simulink model "MOBATSim"  (R2020b)
settings: Solver=FixedStepAuto  StartTime=0.0  StopTime=Sim_t  FixedStep=0.005  MinStep=0.01  RelTol=1e-2
undefined symbols (not defined in the file): FIBlock, FIBlockLib, meters, Sim_Ts, Vehicle_id, Vehicles
libraries: simulink x31, robotalgslib x11, drivingvehiclecontroller x11, mpcadaslib x1, pid_lib x1
(part 2 of 6)

== system MOBATSim/Vehicle Model 3 ==
  note: Perception
  note: Decision-Making
  note: Control
  Behavioural Planner : MATLABSystem  System=VehicleDrivingMode  Vehicle_id=Vehicle_id  SimulateUsing=Interpreted execution
      mask Type: VehicleDrivingMode
      mask Display:
      | image('MOBATSIM-Icon-Set_7- Behavioural Planner.png');
      | port_label('input',1,'vehicleDetected');
      | port_label('output',1,'SpeedReference');
      | port_label('output',2,'DistanceReference');
      | port_label('output',3,'LeadSpeed');
      | port_label('output',4,'DrivingMode');
      | port_label('output',5,'Dist2Stop');
      | port_label('output',6,'laneChange');
  Longitudinal and Lateral Controllers : Subsystem
  Safety Filter : Subsystem
  Transform to MOBATSim Coordinates : Subsystem
  Vehicle Model - Kinematic 3DOF Single Track : Subsystem  mask{Vehicle_id=Vehicle_id}
      mask prompts: Vehicle_id "Vehicle ID"
      mask Display: image('MOBATSIM-Icon-Set_13- VehicleModel.png'); % Use "Edit Image" on toolstrip to change.
  Vehicle Path Planner : MATLABSystem  System=VehiclePathPlanner_Astar  Vehicle_id=Vehicle_id  SimulateUsing=Interpreted execution
      mask Type: VehiclePathPlanner_Astar
      mask Display:
      | image('MOBATSIM-Icon-Set_8- Navigation.png');
      | port_label('input',1,'CommunicationIDs');
      | port_label('output',1,'waypointReached');
  Vehicle Sensors : MATLABSystem  System=VehicleSensors  Vehicle_id=Vehicle_id  Tsample=Sim_Ts  OffsetTime=0  SimulateUsing=Interpreted execution
      mask Type: VehicleSensors
      mask Display:
      | image('MOBATSIM-Icon-Set_4- Sensor.png');
      | port_label('output',1,'V2VcommIDs');
      | port_label('output',2,'vehicleDetected');
  Vehicle V2I Output : MATLABSystem  System=VehicleV2I_Out  Vehicle_id=Vehicle_id  SimulateUsing=Interpreted execution
      mask Type: VehicleV2I_Out
      mask Display:
      | image('MOBATSIM-Icon-Set_6- V2l.png');
      | port_label('input',1,'waypointReached');
      | port_label('output',1,'V2Idata');
  Position : Outport  VectorParamsAs1DForOutWhenUnconnected=off
  Orientation : Outport  Port=2  VectorParamsAs1DForOutWhenUnconnected=off
  Speed : Outport  Port=3  VectorParamsAs1DForOutWhenUnconnected=off
  V_Network_Out : Outport  Port=4  VectorParamsAs1DForOutWhenUnconnected=off
  wires:
  Vehicle Path Planner/1 -> Vehicle V2I Output/1
  Vehicle Sensors/1 -> Vehicle Path Planner/1
  Vehicle V2I Output/1 -> V_Network_Out/1
  Vehicle Sensors/2 -> Behavioural Planner/1
  Behavioural Planner/1 -> Longitudinal and Lateral Controllers/1(Speed Reference)
  Behavioural Planner/2 -> Longitudinal and Lateral Controllers/2(Inter Vehicular Distance)
  Behavioural Planner/3 -> Longitudinal and Lateral Controllers/3(Lead Speed)
  Behavioural Planner/4 -> Longitudinal and Lateral Controllers/4(drivingMode)
  Behavioural Planner/5 -> Longitudinal and Lateral Controllers/5(Dist2Stop)
  Transform to MOBATSim Coordinates/1(Position) -> Position/1
  Transform to MOBATSim Coordinates/2(Orientation) -> Orientation/1
  Vehicle Model - Kinematic 3DOF Single Track/2(xdot) -> Longitudinal and Lateral Controllers/7(Actual Speed), Speed/1
  Vehicle Model - Kinematic 3DOF Single Track/1(Pose) -> Longitudinal and Lateral Controllers/8(Actual Pose), Transform to MOBATSim Coordinates/1(Pose)
  Longitudinal and Lateral Controllers/1(ref Acc) -> Safety Filter/1(Reference Acceleration)
  Longitudinal and Lateral Controllers/2(ref Steering) -> Safety Filter/2(Reference Steering Angle)
  Safety Filter/1(Steering Angle Cmd) -> Vehicle Model - Kinematic 3DOF Single Track/1(WhlAngF)
  Safety Filter/2(Speed_input) -> Vehicle Model - Kinematic 3DOF Single Track/2(xdotin)
  Behavioural Planner/6 -> Longitudinal and Lateral Controllers/6(laneChange)

== system MOBATSim/Vehicle Model 4 ==
  note: Perception
  note: Decision-Making
  note: Control
  Behavioural Planner : MATLABSystem  System=VehicleDrivingMode  Vehicle_id=Vehicle_id  SimulateUsing=Interpreted execution
      mask Type: VehicleDrivingMode
      mask Display:
      | image('MOBATSIM-Icon-Set_7- Behavioural Planner.png');
      | port_label('input',1,'vehicleDetected');
      | port_label('output',1,'SpeedReference');
      | port_label('output',2,'DistanceReference');
      | port_label('output',3,'LeadSpeed');
      | port_label('output',4,'DrivingMode');
      | port_label('output',5,'Dist2Stop');
      | port_label('output',6,'laneChange');
  Longitudinal and Lateral Controllers : Subsystem
  Safety Filter : Subsystem
  Transform to MOBATSim Coordinates : Subsystem
  Vehicle Model - Kinematic 3DOF Single Track : Subsystem  mask{Vehicle_id=Vehicle_id}
      mask prompts: Vehicle_id "Vehicle ID"
      mask Display: image('MOBATSIM-Icon-Set_13- VehicleModel.png'); % Use "Edit Image" on toolstrip to change.
  Vehicle Path Planner : MATLABSystem  System=VehiclePathPlanner_Astar  Vehicle_id=Vehicle_id  SimulateUsing=Interpreted execution
      mask Type: VehiclePathPlanner_Astar
      mask Display:
      | image('MOBATSIM-Icon-Set_8- Navigation.png');
      | port_label('input',1,'CommunicationIDs');
      | port_label('output',1,'waypointReached');
  Vehicle Sensors : MATLABSystem  System=VehicleSensors  Vehicle_id=Vehicle_id  Tsample=Sim_Ts  OffsetTime=0  SimulateUsing=Interpreted execution
      mask Type: VehicleSensors
      mask Display:
      | image('MOBATSIM-Icon-Set_4- Sensor.png');
      | port_label('output',1,'V2VcommIDs');
      | port_label('output',2,'vehicleDetected');
  Vehicle V2I Output : MATLABSystem  System=VehicleV2I_Out  Vehicle_id=Vehicle_id  SimulateUsing=Interpreted execution
      mask Type: VehicleV2I_Out
      mask Display:
      | image('MOBATSIM-Icon-Set_6- V2l.png');
      | port_label('input',1,'waypointReached');
      | port_label('output',1,'V2Idata');
  Position : Outport  VectorParamsAs1DForOutWhenUnconnected=off
  Orientation : Outport  Port=2  VectorParamsAs1DForOutWhenUnconnected=off
  Speed : Outport  Port=3  VectorParamsAs1DForOutWhenUnconnected=off
  V_Network_Out : Outport  Port=4  VectorParamsAs1DForOutWhenUnconnected=off
  wires:
  Vehicle Path Planner/1 -> Vehicle V2I Output/1
  Vehicle Sensors/1 -> Vehicle Path Planner/1
  Vehicle V2I Output/1 -> V_Network_Out/1
  Vehicle Sensors/2 -> Behavioural Planner/1
  Behavioural Planner/1 -> Longitudinal and Lateral Controllers/1(Speed Reference)
  Behavioural Planner/2 -> Longitudinal and Lateral Controllers/2(Inter Vehicular Distance)
  Behavioural Planner/3 -> Longitudinal and Lateral Controllers/3(Lead Speed)
  Behavioural Planner/4 -> Longitudinal and Lateral Controllers/4(drivingMode)
  Behavioural Planner/5 -> Longitudinal and Lateral Controllers/5(Dist2Stop)
  Transform to MOBATSim Coordinates/1(Position) -> Position/1
  Transform to MOBATSim Coordinates/2(Orientation) -> Orientation/1
  Vehicle Model - Kinematic 3DOF Single Track/2(xdot) -> Longitudinal and Lateral Controllers/7(Actual Speed), Speed/1
  Vehicle Model - Kinematic 3DOF Single Track/1(Pose) -> Longitudinal and Lateral Controllers/8(Actual Pose), Transform to MOBATSim Coordinates/1(Pose)
  Longitudinal and Lateral Controllers/1(ref Acc) -> Safety Filter/1(Reference Acceleration)
  Longitudinal and Lateral Controllers/2(ref Steering) -> Safety Filter/2(Reference Steering Angle)
  Safety Filter/1(Steering Angle Cmd) -> Vehicle Model - Kinematic 3DOF Single Track/1(WhlAngF)
  Safety Filter/2(Speed_input) -> Vehicle Model - Kinematic 3DOF Single Track/2(xdotin)
  Behavioural Planner/6 -> Longitudinal and Lateral Controllers/6(laneChange)

== system MOBATSim/Vehicle Model 5 ==
  note: Perception
  note: Decision-Making
  note: Control
  Behavioural Planner : MATLABSystem  System=VehicleDrivingMode  Vehicle_id=Vehicle_id  SimulateUsing=Interpreted execution
      mask Type: VehicleDrivingMode
      mask Display:
      | image('MOBATSIM-Icon-Set_7- Behavioural Planner.png');
      | port_label('input',1,'vehicleDetected');
      | port_label('output',1,'SpeedReference');
      | port_label('output',2,'DistanceReference');
      | port_label('output',3,'LeadSpeed');
      | port_label('output',4,'DrivingMode');
      | port_label('output',5,'Dist2Stop');
      | port_label('output',6,'laneChange');
  Longitudinal and Lateral Controllers : Subsystem
  Safety Filter : Subsystem
  Transform to MOBATSim Coordinates : Subsystem
  Vehicle Model - Kinematic 3DOF Single Track : Subsystem  mask{Vehicle_id=Vehicle_id}
      mask prompts: Vehicle_id "Vehicle ID"
      mask Display: image('MOBATSIM-Icon-Set_13- VehicleModel.png'); % Use "Edit Image" on toolstrip to change.
  Vehicle Path Planner : MATLABSystem  System=VehiclePathPlanner_Astar  Vehicle_id=Vehicle_id  SimulateUsing=Interpreted execution
      mask Type: VehiclePathPlanner_Astar
      mask Display:
      | image('MOBATSIM-Icon-Set_8- Navigation.png');
      | port_label('input',1,'CommunicationIDs');
      | port_label('output',1,'waypointReached');
  Vehicle Sensors : MATLABSystem  System=VehicleSensors  Vehicle_id=Vehicle_id  Tsample=Sim_Ts  OffsetTime=0  SimulateUsing=Interpreted execution
      mask Type: VehicleSensors
      mask Display:
      | image('MOBATSIM-Icon-Set_4- Sensor.png');
      | port_label('output',1,'V2VcommIDs');
      | port_label('output',2,'vehicleDetected');
  Vehicle V2I Output : MATLABSystem  System=VehicleV2I_Out  Vehicle_id=Vehicle_id  SimulateUsing=Interpreted execution
      mask Type: VehicleV2I_Out
      mask Display:
      | image('MOBATSIM-Icon-Set_6- V2l.png');
      | port_label('input',1,'waypointReached');
      | port_label('output',1,'V2Idata');
  Position : Outport  VectorParamsAs1DForOutWhenUnconnected=off
  Orientation : Outport  Port=2  VectorParamsAs1DForOutWhenUnconnected=off
  Speed : Outport  Port=3  VectorParamsAs1DForOutWhenUnconnected=off
  V_Network_Out : Outport  Port=4  VectorParamsAs1DForOutWhenUnconnected=off
  wires:
  Vehicle Path Planner/1 -> Vehicle V2I Output/1
  Vehicle Sensors/1 -> Vehicle Path Planner/1
  Vehicle V2I Output/1 -> V_Network_Out/1
  Vehicle Sensors/2 -> Behavioural Planner/1
  Behavioural Planner/1 -> Longitudinal and Lateral Controllers/1(Speed Reference)
  Behavioural Planner/2 -> Longitudinal and Lateral Controllers/2(Inter Vehicular Distance)
  Behavioural Planner/3 -> Longitudinal and Lateral Controllers/3(Lead Speed)
  Behavioural Planner/4 -> Longitudinal and Lateral Controllers/4(drivingMode)
  Behavioural Planner/5 -> Longitudinal and Lateral Controllers/5(Dist2Stop)
  Transform to MOBATSim Coordinates/1(Position) -> Position/1
  Transform to MOBATSim Coordinates/2(Orientation) -> Orientation/1
  Vehicle Model - Kinematic 3DOF Single Track/2(xdot) -> Longitudinal and Lateral Controllers/7(Actual Speed), Speed/1
  Vehicle Model - Kinematic 3DOF Single Track/1(Pose) -> Longitudinal and Lateral Controllers/8(Actual Pose), Transform to MOBATSim Coordinates/1(Pose)
  Longitudinal and Lateral Controllers/1(ref Acc) -> Safety Filter/1(Reference Acceleration)
  Longitudinal and Lateral Controllers/2(ref Steering) -> Safety Filter/2(Reference Steering Angle)
  Safety Filter/1(Steering Angle Cmd) -> Vehicle Model - Kinematic 3DOF Single Track/1(WhlAngF)
  Safety Filter/2(Speed_input) -> Vehicle Model - Kinematic 3DOF Single Track/2(xdotin)
  Behavioural Planner/6 -> Longitudinal and Lateral Controllers/6(laneChange)

== system MOBATSim/Vehicle Model 6 ==
  note: Perception
  note: Decision-Making
  note: Control
  Behavioural Planner : MATLABSystem  System=VehicleDrivingMode  Vehicle_id=Vehicle_id  SimulateUsing=Interpreted execution
      mask Type: VehicleDrivingMode
      mask Display:
      | image('MOBATSIM-Icon-Set_7- Behavioural Planner.png');
      | port_label('input',1,'vehicleDetected');
      | port_label('output',1,'SpeedReference');
      | port_label('output',2,'DistanceReference');
      | port_label('output',3,'LeadSpeed');
      | port_label('output',4,'DrivingMode');
      | port_label('output',5,'Dist2Stop');
      | port_label('output',6,'laneChange');
  FIBlock : Subsystem  AncestorBlock=FIBlockLib/FIBlock  TreatAsAtomicUnit=on  mask(Fault Injector Block){FIBlockName=1, FInjEnable=on, FaultType=Noise, FaultValue=20, FaultEvent=Deterministic, EventValue=0, FaultEffect=Constant time, EffectValue=4.2}
      mask prompts: FIBlockName "Number of the FI block instance (e.i. 'name' of the fault injector)"; FInjEnable "Turn on the fault injection for this block"; FaultType "Fault type"; FaultValue "Fault value (boundaries, %)"; FaultEvent "Fault injection method"; EventValue "Event value (s)"; FaultEffect "Fault injection effect"; EffectValue "Effect value (s)"
      mask help:
      | This block allows to conduct a fault injection experiment (refer to help if needed).
      | Specify:
      | - name of the block instance.
      | - type of fault: Stuck-at, Package drop, Bias/Offset, Bit flips, Time delay, Noise.
      | - fault event: Failure probability, Mean Time to Failure, Failure Rate Distribution, Deterministic.
      | - fault effect: Once, Constant time, Infinite time, Mean Time to Repair.
      mask init: same as MOBATSim/Vehicle Model 2/FIBlock1
      mask Help:
      | Failure rate distribution is not supported yet!
      | Bit flips, Time delay, and Noise faults may have some bugs :D
      | In different FIBlock instances, the 'name' of the block in GUI must be different (must be an integer number).
      | 
      | Please refer to a comprehensive article regarding the FIBLock: https://flatag.tech/fiblock.html
      | Please cite as: "Fabarisov, T. et al. "Model-based Fault Injection Experiments for the Safety Analysis of Exoskeleton System." Proceedings of the 30th European Safety and Reliability Conference and the 15th Probabilistic Safety Assessment and Management Conference, 2020."
      | 
      | This block allows to conduct a fault injection experiment.
      | Specify:
      | 1) number of the block instance (e.i. 'name' of the fault injector, name shall be unique).
      | 
      | 2) type of fault:
      | - Stuck-at. The block output stays constant, preserving the latest correct value before the error occurrence.
      | - Package drop. The correct output is replaced by the specified Value, emulating a package drop.
      | - Bias/Offset . The defined positive or negative Bias value is added to the block output.
      | - Noise. A random noise value is added. The Boundaries are defined as the percentage of the correct value.
      | - Time delay. A delay is introduced into the signal. During the delay the value is zero.
      | - Bit flips. The defined Number of bits are inverted in the binary representation of the correct value.
      | 
      | 3) fault event:
      | - Failure probability. Errors are injected based on the constant Failure probability for each execution of the block function.
      | - Mean Time to Failure. Errors are injected according to the specified MTTF. Normal distribution.
      | - Deterministic. Уrrors are injected at specific time step.
      | 
      | 4) fault effect:
      | - Once. An error appears only one time during a simulation.
      | - Constant time. The block produces erroneous output during the specified Time period.
      | - Infinite time. The block produces erroneous output until the end of the simulation.
      | - Mean Time to Repair. Normally distributed MTTR regulates the time of the error effect.
      | 
      | FIBlock also provide, what we call, a chained fault injection.
      | Second output of the FIBlock emits a trigger flag.
      | This output signal could be connected to the second input of the FIBlock.
      | In case of the fault injection, this signal will force trigger fault injectionin second FIBlock.
      | 
      | FIBlock supports a base Workspace variables as input in the GUI parameters.
      | 
      | Made By Tagir Fabarisov, TU Dresden 2020
      mask TypeOptions FaultType: Stuck-at | Package drop | Bias/Offset | Bit flips | Time delay | Noise
      mask TypeOptions FaultEvent: Failure probability | Mean Time To Failure | Deterministic
      mask TypeOptions FaultEffect: Once | Constant time | Infinite time | Mean Time To Repair
      mask DialogControl FInjEnable Tooltip: If ticked, then this FIBlock will inject faults
      mask DialogControl Container8 Prompt: Fault type
      mask DialogControl FaultType Tooltip: Specify a type of fault that will be injected
      mask DialogControl FaultTypeDesc Prompt: A random noise value is added. The Boundaries are defined as the percentage of the correct value.
      mask DialogControl Container3 Prompt: Fault injection method
      mask DialogControl Container6 Prompt: Event
      mask DialogControl FaultEvent Tooltip: Specify when fault will be injected
      mask DialogControl FaultEventDesc Prompt: Errors are injected at the specified time
      mask DialogControl Container7 Prompt: Effect
      mask DialogControl FaultEffect Tooltip: Specify how long fault will be injected
      mask DialogControl FaultEffectDesc Prompt: The block produces erroneous output during the specified Time period.
      mask Display:
      | warning off;
      | color('red');
      | a = FaultType;
      | if a == "Sensor: Stuck-at fault"
      |     color('black');
      |     x = linspace(-pi,pi);
      |     y = sin(x);
      |     plot(x,y);
      |     color('red');
      |     disp('        ↯');
      |     x = [-0.7 2];
      |     y = [-0.7 -0.7];
      |     plot(x,y);
      | elseif a == "Network: Package drop"
      |     color('black');
      |     x = linspace(-pi,pi);
      |     y = sin(x);
      |     plot(x,y);
      |     color('red');
      |     disp('        ↯');
      |     x = [-0.7 -0.7];
      |     y = [-0.7 0];
      |     plot(x,y);
      |     x = [-0.7 1];
      |     y = [0 0];
      |     plot(x,y);
      | elseif a == "Sensor: Offset"
      |     color('black');
      |     x1 = linspace(-pi,pi);
      |     y1 = sin(x1)-0.5;
      |     plot(x1,y1);
      |     color('red');
      |     disp('        ↯');
      |     x2 = linspace(0,pi);
      |     y2 = sin(x2);
      |     plot(x2,y2);
      |     x = [0 0];
      |     y = [-0.5 0];
      |     plot(x,y);
      | elseif a == "Hardware: Bit flips"
      |     color('black');
      |     disp('10101010');
      |     color('red');
      |     disp('    0↯');
      | elseif a == "Network: Time delay"
      |     color('black');
      |     x1 = linspace(-pi,pi);
      |     y1 = sin(x1);
      |     plot(x1,y1);
      |     color('red');
      |     disp('        ↯');
      |     x2 = linspace(0,pi);
      |     y2 = sin(x2-0.5);
      |     plot(x2,y2);
      |     x = [0 -0.4];
      |     y = [-0.5 -0.5];
      |     plot(x,y);
      | elseif a == "Sensor: Noise"
      |     color('black');
      |     x1 = linspace(-pi,pi);
      |     y1 = sin(x1);
      |     plot(x1,y1);
      |     color('red');
      |     disp('        ↯');
      |     x = linspace(-pi/8,pi/8,10);
      |     y = sin(x);
      |     for yc = 1:length(y)
      |         d = randi([-2,2])/5;
      |         y(yc) = y(yc) + d;
      |     end
      |     plot(x,y);
      | else
      |     color('red');
      |     disp('Set up Fault Injector!');
      | %Bit flips
      | %Time delay
      | %Noise
      | end
      | warning on;
  FIBlock1 : Subsystem  AncestorBlock=FIBlockLib/FIBlock  TreatAsAtomicUnit=on  mask(Fault Injector Block){FIBlockName=2, FInjEnable=on, FaultType=Noise, FaultValue=20, FaultEvent=Deterministic, EventValue=0, FaultEffect=Constant time, EffectValue=4.2}
      mask prompts: FIBlockName "Number of the FI block instance (e.i. 'name' of the fault injector)"; FInjEnable "Turn on the fault injection for this block"; FaultType "Fault type"; FaultValue "Fault value (boundaries, %)"; FaultEvent "Fault injection method"; EventValue "Event value (s)"; FaultEffect "Fault injection effect"; EffectValue "Effect value (s)"
      mask help:
      | This block allows to conduct a fault injection experiment (refer to help if needed).
      | Specify:
      | - name of the block instance.
      | - type of fault: Stuck-at, Package drop, Bias/Offset, Bit flips, Time delay, Noise.
      | - fault event: Failure probability, Mean Time to Failure, Failure Rate Distribution, Deterministic.
      | - fault effect: Once, Constant time, Infinite time, Mean Time to Repair.
      mask init: same as MOBATSim/Vehicle Model 2/FIBlock1
      mask Help:
      | Failure rate distribution is not supported yet!
      | Bit flips, Time delay, and Noise faults may have some bugs :D
      | In different FIBlock instances, the 'name' of the block in GUI must be different (must be an integer number).
      | 
      | Please refer to a comprehensive article regarding the FIBLock: https://flatag.tech/fiblock.html
      | Please cite as: "Fabarisov, T. et al. "Model-based Fault Injection Experiments for the Safety Analysis of Exoskeleton System." Proceedings of the 30th European Safety and Reliability Conference and the 15th Probabilistic Safety Assessment and Management Conference, 2020."
      | 
      | This block allows to conduct a fault injection experiment.
      | Specify:
      | 1) number of the block instance (e.i. 'name' of the fault injector, name shall be unique).
      | 
      | 2) type of fault:
      | - Stuck-at. The block output stays constant, preserving the latest correct value before the error occurrence.
      | - Package drop. The correct output is replaced by the specified Value, emulating a package drop.
      | - Bias/Offset . The defined positive or negative Bias value is added to the block output.
      | - Noise. A random noise value is added. The Boundaries are defined as the percentage of the correct value.
      | - Time delay. A delay is introduced into the signal. During the delay the value is zero.
      | - Bit flips. The defined Number of bits are inverted in the binary representation of the correct value.
      | 
      | 3) fault event:
      | - Failure probability. Errors are injected based on the constant Failure probability for each execution of the block function.
      | - Mean Time to Failure. Errors are injected according to the specified MTTF. Normal distribution.
      | - Deterministic. Уrrors are injected at specific time step.
      | 
      | 4) fault effect:
      | - Once. An error appears only one time during a simulation.
      | - Constant time. The block produces erroneous output during the specified Time period.
      | - Infinite time. The block produces erroneous output until the end of the simulation.
      | - Mean Time to Repair. Normally distributed MTTR regulates the time of the error effect.
      | 
      | FIBlock also provide, what we call, a chained fault injection.
      | Second output of the FIBlock emits a trigger flag.
      | This output signal could be connected to the second input of the FIBlock.
      | In case of the fault injection, this signal will force trigger fault injectionin second FIBlock.
      | 
      | FIBlock supports a base Workspace variables as input in the GUI parameters.
      | 
      | Made By Tagir Fabarisov, TU Dresden 2020
      mask TypeOptions FaultType: Stuck-at | Package drop | Bias/Offset | Bit flips | Time delay | Noise
      mask TypeOptions FaultEvent: Failure probability | Mean Time To Failure | Deterministic
      mask TypeOptions FaultEffect: Once | Constant time | Infinite time | Mean Time To Repair
      mask DialogControl FInjEnable Tooltip: If ticked, then this FIBlock will inject faults
      mask DialogControl Container8 Prompt: Fault type
      mask DialogControl FaultType Tooltip: Specify a type of fault that will be injected
      mask DialogControl FaultTypeDesc Prompt: A random noise value is added. The Boundaries are defined as the percentage of the correct value.
      mask DialogControl Container3 Prompt: Fault injection method
      mask DialogControl Container6 Prompt: Event
      mask DialogControl FaultEvent Tooltip: Specify when fault will be injected
      mask DialogControl FaultEventDesc Prompt: Errors are injected at the specified time
      mask DialogControl Container7 Prompt: Effect
      mask DialogControl FaultEffect Tooltip: Specify how long fault will be injected
      mask DialogControl FaultEffectDesc Prompt: The block produces erroneous output during the specified Time period.
      mask Display:
      | warning off;
      | color('red');
      | a = FaultType;
      | if a == "Sensor: Stuck-at fault"
      |     color('black');
      |     x = linspace(-pi,pi);
      |     y = sin(x);
      |     plot(x,y);
      |     color('red');
      |     disp('        ↯');
      |     x = [-0.7 2];
      |     y = [-0.7 -0.7];
      |     plot(x,y);
      | elseif a == "Network: Package drop"
      |     color('black');
      |     x = linspace(-pi,pi);
      |     y = sin(x);
      |     plot(x,y);
      |     color('red');
      |     disp('        ↯');
      |     x = [-0.7 -0.7];
      |     y = [-0.7 0];
      |     plot(x,y);
      |     x = [-0.7 1];
      |     y = [0 0];
      |     plot(x,y);
      | elseif a == "Sensor: Offset"
      |     color('black');
      |     x1 = linspace(-pi,pi);
      |     y1 = sin(x1)-0.5;
      |     plot(x1,y1);
      |     color('red');
      |     disp('        ↯');
      |     x2 = linspace(0,pi);
      |     y2 = sin(x2);
      |     plot(x2,y2);
      |     x = [0 0];
      |     y = [-0.5 0];
      |     plot(x,y);
      | elseif a == "Hardware: Bit flips"
      |     color('black');
      |     disp('10101010');
      |     color('red');
      |     disp('    0↯');
      | elseif a == "Network: Time delay"
      |     color('black');
      |     x1 = linspace(-pi,pi);
      |     y1 = sin(x1);
      |     plot(x1,y1);
      |     color('red');
      |     disp('        ↯');
      |     x2 = linspace(0,pi);
      |     y2 = sin(x2-0.5);
      |     plot(x2,y2);
      |     x = [0 -0.4];
      |     y = [-0.5 -0.5];
      |     plot(x,y);
      | elseif a == "Sensor: Noise"
      |     color('black');
      |     x1 = linspace(-pi,pi);
      |     y1 = sin(x1);
      |     plot(x1,y1);
      |     color('red');
      |     disp('        ↯');
      |     x = linspace(-pi/8,pi/8,10);
      |     y = sin(x);
      |     for yc = 1:length(y)
      |         d = randi([-2,2])/5;
      |         y(yc) = y(yc) + d;
      |     end
      |     plot(x,y);
      | else
      |     color('red');
      |     disp('Set up Fault Injector!');
      | %Bit flips
      | %Time delay
      | %Noise
      | end
      | warning on;
  Longitudinal and Lateral Controllers : Subsystem
  Pulse Generator : DiscretePulseGenerator  PulseType=Time based  Period=10  PulseWidth=5
  Pulse Generator1 : DiscretePulseGenerator  PulseType=Time based  Period=10  PulseWidth=5
  Safety Filter : Subsystem
  Transform to MOBATSim Coordinates : Subsystem
  Vehicle Model - Kinematic 3DOF Single Track : Subsystem  mask{Vehicle_id=Vehicle_id}
      mask prompts: Vehicle_id "Vehicle ID"
      mask Display: image('MOBATSIM-Icon-Set_13- VehicleModel.png'); % Use "Edit Image" on toolstrip to change.
  Vehicle Path Planner : MATLABSystem  System=VehiclePathPlanner_Astar  Vehicle_id=Vehicle_id  SimulateUsing=Interpreted execution
      mask Type: VehiclePathPlanner_Astar
      mask Display:
      | image('MOBATSIM-Icon-Set_8- Navigation.png');
      | port_label('input',1,'CommunicationIDs');
      | port_label('output',1,'waypointReached');
  Vehicle Sensors : MATLABSystem  System=VehicleSensors  Vehicle_id=Vehicle_id  Tsample=Sim_Ts  OffsetTime=0  SimulateUsing=Interpreted execution
      mask Type: VehicleSensors
      mask Display:
      | image('MOBATSIM-Icon-Set_4- Sensor.png');
      | port_label('output',1,'V2VcommIDs');
      | port_label('output',2,'vehicleDetected');
  Vehicle V2I Output : MATLABSystem  System=VehicleV2I_Out  Vehicle_id=Vehicle_id  SimulateUsing=Interpreted execution
      mask Type: VehicleV2I_Out
      mask Display:
      | image('MOBATSIM-Icon-Set_6- V2l.png');
      | port_label('input',1,'waypointReached');
      | port_label('output',1,'V2Idata');
  Position : Outport  VectorParamsAs1DForOutWhenUnconnected=off
  Orientation : Outport  Port=2  VectorParamsAs1DForOutWhenUnconnected=off
  Speed : Outport  Port=3  VectorParamsAs1DForOutWhenUnconnected=off
  V_Network_Out : Outport  Port=4  VectorParamsAs1DForOutWhenUnconnected=off
  wires:
  Vehicle Path Planner/1 -> Vehicle V2I Output/1
  Vehicle Sensors/1 -> Vehicle Path Planner/1
  Vehicle V2I Output/1 -> V_Network_Out/1
  Vehicle Sensors/2 -> Behavioural Planner/1
  Behavioural Planner/3 -> Longitudinal and Lateral Controllers/3(Lead Speed)
  Behavioural Planner/4 -> Longitudinal and Lateral Controllers/4(drivingMode)
  Behavioural Planner/5 -> Longitudinal and Lateral Controllers/5(Dist2Stop)
  Transform to MOBATSim Coordinates/1(Position) -> Position/1
  Transform to MOBATSim Coordinates/2(Orientation) -> Orientation/1
  Vehicle Model - Kinematic 3DOF Single Track/2(xdot) -> Longitudinal and Lateral Controllers/7(Actual Speed), Speed/1
  Vehicle Model - Kinematic 3DOF Single Track/1(Pose) -> Longitudinal and Lateral Controllers/8(Actual Pose), Transform to MOBATSim Coordinates/1(Pose)
  Longitudinal and Lateral Controllers/1(ref Acc) -> Safety Filter/1(Reference Acceleration)
  Longitudinal and Lateral Controllers/2(ref Steering) -> Safety Filter/2(Reference Steering Angle)
  Safety Filter/1(Steering Angle Cmd) -> Vehicle Model - Kinematic 3DOF Single Track/1(WhlAngF)
  Safety Filter/2(Speed_input) -> Vehicle Model - Kinematic 3DOF Single Track/2(xdotin)
  Behavioural Planner/6 -> Longitudinal and Lateral Controllers/6(laneChange)
  Behavioural Planner/1 -> FIBlock/1(Idata)
  FIBlock/1(Fdata) -> Longitudinal and Lateral Controllers/1(Speed Reference)
  Behavioural Planner/2 -> FIBlock1/1(Idata)
  FIBlock1/1(Fdata) -> Longitudinal and Lateral Controllers/2(Inter Vehicular Distance)
  Pulse Generator1/1 -> FIBlock/2(Iflag)
  Pulse Generator/1 -> FIBlock1/2(Iflag)

== system MOBATSim/Vehicle Model 7 ==
  note: Perception
  note: Decision-Making
  note: Control
  Behavioural Planner : MATLABSystem  System=VehicleDrivingMode  Vehicle_id=Vehicle_id  SimulateUsing=Interpreted execution
      mask Type: VehicleDrivingMode
      mask Display:
      | image('MOBATSIM-Icon-Set_7- Behavioural Planner.png');
      | port_label('input',1,'vehicleDetected');
      | port_label('output',1,'SpeedReference');
      | port_label('output',2,'DistanceReference');
      | port_label('output',3,'LeadSpeed');
      | port_label('output',4,'DrivingMode');
      | port_label('output',5,'Dist2Stop');
      | port_label('output',6,'laneChange');
  Longitudinal and Lateral Controllers : Subsystem
  Safety Filter : Subsystem
  Transform to MOBATSim Coordinates : Subsystem
  Vehicle Model - Kinematic 3DOF Single Track : Subsystem  mask{Vehicle_id=Vehicle_id}
      mask prompts: Vehicle_id "Vehicle ID"
      mask Display: image('MOBATSIM-Icon-Set_13- VehicleModel.png'); % Use "Edit Image" on toolstrip to change.
  Vehicle Path Planner : MATLABSystem  System=VehiclePathPlanner_Astar  Vehicle_id=Vehicle_id  SimulateUsing=Interpreted execution
      mask Type: VehiclePathPlanner_Astar
      mask Display:
      | image('MOBATSIM-Icon-Set_8- Navigation.png');
      | port_label('input',1,'CommunicationIDs');
      | port_label('output',1,'waypointReached');
  Vehicle Sensors : MATLABSystem  System=VehicleSensors  Vehicle_id=Vehicle_id  Tsample=Sim_Ts  OffsetTime=0  SimulateUsing=Interpreted execution
      mask Type: VehicleSensors
      mask Display:
      | image('MOBATSIM-Icon-Set_4- Sensor.png');
      | port_label('output',1,'V2VcommIDs');
      | port_label('output',2,'vehicleDetected');
  Vehicle V2I Output : MATLABSystem  System=VehicleV2I_Out  Vehicle_id=Vehicle_id  SimulateUsing=Interpreted execution
      mask Type: VehicleV2I_Out
      mask Display:
      | image('MOBATSIM-Icon-Set_6- V2l.png');
      | port_label('input',1,'waypointReached');
      | port_label('output',1,'V2Idata');
  Position : Outport  VectorParamsAs1DForOutWhenUnconnected=off
  Orientation : Outport  Port=2  VectorParamsAs1DForOutWhenUnconnected=off
  Speed : Outport  Port=3  VectorParamsAs1DForOutWhenUnconnected=off
  V_Network_Out : Outport  Port=4  VectorParamsAs1DForOutWhenUnconnected=off
  wires:
  Vehicle Path Planner/1 -> Vehicle V2I Output/1
  Vehicle Sensors/1 -> Vehicle Path Planner/1
  Vehicle V2I Output/1 -> V_Network_Out/1
  Vehicle Sensors/2 -> Behavioural Planner/1
  Behavioural Planner/1 -> Longitudinal and Lateral Controllers/1(Speed Reference)
  Behavioural Planner/2 -> Longitudinal and Lateral Controllers/2(Inter Vehicular Distance)
  Behavioural Planner/3 -> Longitudinal and Lateral Controllers/3(Lead Speed)
  Behavioural Planner/4 -> Longitudinal and Lateral Controllers/4(drivingMode)
  Behavioural Planner/5 -> Longitudinal and Lateral Controllers/5(Dist2Stop)
  Transform to MOBATSim Coordinates/1(Position) -> Position/1
  Transform to MOBATSim Coordinates/2(Orientation) -> Orientation/1
  Vehicle Model - Kinematic 3DOF Single Track/2(xdot) -> Longitudinal and Lateral Controllers/7(Actual Speed), Speed/1
  Vehicle Model - Kinematic 3DOF Single Track/1(Pose) -> Longitudinal and Lateral Controllers/8(Actual Pose), Transform to MOBATSim Coordinates/1(Pose)
  Longitudinal and Lateral Controllers/1(ref Acc) -> Safety Filter/1(Reference Acceleration)
  Longitudinal and Lateral Controllers/2(ref Steering) -> Safety Filter/2(Reference Steering Angle)
  Safety Filter/1(Steering Angle Cmd) -> Vehicle Model - Kinematic 3DOF Single Track/1(WhlAngF)
  Safety Filter/2(Speed_input) -> Vehicle Model - Kinematic 3DOF Single Track/2(xdotin)
  Behavioural Planner/6 -> Longitudinal and Lateral Controllers/6(laneChange)

== system MOBATSim/Vehicle Model 8 ==
  note: Perception
  note: Decision-Making
  note: Control
  Behavioural Planner : MATLABSystem  System=VehicleDrivingMode  Vehicle_id=Vehicle_id  SimulateUsing=Interpreted execution
      mask Type: VehicleDrivingMode
      mask Display:
      | image('MOBATSIM-Icon-Set_7- Behavioural Planner.png');
      | port_label('input',1,'vehicleDetected');
      | port_label('output',1,'SpeedReference');
      | port_label('output',2,'DistanceReference');
      | port_label('output',3,'LeadSpeed');
      | port_label('output',4,'DrivingMode');
      | port_label('output',5,'Dist2Stop');
      | port_label('output',6,'laneChange');
  Longitudinal and Lateral Controllers : Subsystem
  Safety Filter : Subsystem
  Transform to MOBATSim Coordinates : Subsystem
  Vehicle Model - Kinematic 3DOF Single Track : Subsystem  mask{Vehicle_id=Vehicle_id}
      mask prompts: Vehicle_id "Vehicle ID"
      mask Display: image('MOBATSIM-Icon-Set_13- VehicleModel.png'); % Use "Edit Image" on toolstrip to change.
  Vehicle Path Planner : MATLABSystem  System=VehiclePathPlanner_Astar  Vehicle_id=Vehicle_id  SimulateUsing=Interpreted execution
      mask Type: VehiclePathPlanner_Astar
      mask Display:
      | image('MOBATSIM-Icon-Set_8- Navigation.png');
      | port_label('input',1,'CommunicationIDs');
      | port_label('output',1,'waypointReached');
  Vehicle Sensors : MATLABSystem  System=VehicleSensors  Vehicle_id=Vehicle_id  Tsample=Sim_Ts  OffsetTime=0  SimulateUsing=Interpreted execution
      mask Type: VehicleSensors
      mask Display:
      | image('MOBATSIM-Icon-Set_4- Sensor.png');
      | port_label('output',1,'V2VcommIDs');
      | port_label('output',2,'vehicleDetected');
  Vehicle V2I Output : MATLABSystem  System=VehicleV2I_Out  Vehicle_id=Vehicle_id  SimulateUsing=Interpreted execution
      mask Type: VehicleV2I_Out
      mask Display:
      | image('MOBATSIM-Icon-Set_6- V2l.png');
      | port_label('input',1,'waypointReached');
      | port_label('output',1,'V2Idata');
  Position : Outport  VectorParamsAs1DForOutWhenUnconnected=off
  Orientation : Outport  Port=2  VectorParamsAs1DForOutWhenUnconnected=off
  Speed : Outport  Port=3  VectorParamsAs1DForOutWhenUnconnected=off
  V_Network_Out : Outport  Port=4  VectorParamsAs1DForOutWhenUnconnected=off
  wires:
  Vehicle Path Planner/1 -> Vehicle V2I Output/1
  Vehicle Sensors/1 -> Vehicle Path Planner/1
  Vehicle V2I Output/1 -> V_Network_Out/1
  Vehicle Sensors/2 -> Behavioural Planner/1
  Behavioural Planner/1 -> Longitudinal and Lateral Controllers/1(Speed Reference)
  Behavioural Planner/2 -> Longitudinal and Lateral Controllers/2(Inter Vehicular Distance)
  Behavioural Planner/3 -> Longitudinal and Lateral Controllers/3(Lead Speed)
  Behavioural Planner/4 -> Longitudinal and Lateral Controllers/4(drivingMode)
  Behavioural Planner/5 -> Longitudinal and Lateral Controllers/5(Dist2Stop)
  Transform to MOBATSim Coordinates/1(Position) -> Position/1
  Transform to MOBATSim Coordinates/2(Orientation) -> Orientation/1
  Vehicle Model - Kinematic 3DOF Single Track/2(xdot) -> Longitudinal and Lateral Controllers/7(Actual Speed), Speed/1
  Vehicle Model - Kinematic 3DOF Single Track/1(Pose) -> Longitudinal and Lateral Controllers/8(Actual Pose), Transform to MOBATSim Coordinates/1(Pose)
  Longitudinal and Lateral Controllers/1(ref Acc) -> Safety Filter/1(Reference Acceleration)
  Longitudinal and Lateral Controllers/2(ref Steering) -> Safety Filter/2(Reference Steering Angle)
  Safety Filter/1(Steering Angle Cmd) -> Vehicle Model - Kinematic 3DOF Single Track/1(WhlAngF)
  Safety Filter/2(Speed_input) -> Vehicle Model - Kinematic 3DOF Single Track/2(xdotin)
  Behavioural Planner/6 -> Longitudinal and Lateral Controllers/6(laneChange)

== system MOBATSim/Vehicle Model 9 ==
  note: Perception
  note: Decision-Making
  note: Control
  Behavioural Planner : MATLABSystem  System=VehicleDrivingMode  Vehicle_id=Vehicle_id  SimulateUsing=Interpreted execution
      mask Type: VehicleDrivingMode
      mask Display:
      | image('MOBATSIM-Icon-Set_7- Behavioural Planner.png');
      | port_label('input',1,'vehicleDetected');
      | port_label('output',1,'SpeedReference');
      | port_label('output',2,'DistanceReference');
      | port_label('output',3,'LeadSpeed');
      | port_label('output',4,'DrivingMode');
      | port_label('output',5,'Dist2Stop');
      | port_label('output',6,'laneChange');
  Longitudinal and Lateral Controllers : Subsystem
  Safety Filter : Subsystem
  Transform to MOBATSim Coordinates : Subsystem
  Vehicle Model - Kinematic 3DOF Single Track : Subsystem  mask{Vehicle_id=Vehicle_id}
      mask prompts: Vehicle_id "Vehicle ID"
      mask Display: image('MOBATSIM-Icon-Set_13- VehicleModel.png'); % Use "Edit Image" on toolstrip to change.
  Vehicle Path Planner : MATLABSystem  System=VehiclePathPlanner_Astar  Vehicle_id=Vehicle_id  SimulateUsing=Interpreted execution
      mask Type: VehiclePathPlanner_Astar
      mask Display:
      | image('MOBATSIM-Icon-Set_8- Navigation.png');
      | port_label('input',1,'CommunicationIDs');
      | port_label('output',1,'waypointReached');
  Vehicle Sensors : MATLABSystem  System=VehicleSensors  Vehicle_id=Vehicle_id  Tsample=Sim_Ts  OffsetTime=0  SimulateUsing=Interpreted execution
      mask Type: VehicleSensors
      mask Display:
      | image('MOBATSIM-Icon-Set_4- Sensor.png');
      | port_label('output',1,'V2VcommIDs');
      | port_label('output',2,'vehicleDetected');
  Vehicle V2I Output : MATLABSystem  System=VehicleV2I_Out  Vehicle_id=Vehicle_id  SimulateUsing=Interpreted execution
      mask Type: VehicleV2I_Out
      mask Display:
      | image('MOBATSIM-Icon-Set_6- V2l.png');
      | port_label('input',1,'waypointReached');
      | port_label('output',1,'V2Idata');
  Position : Outport  VectorParamsAs1DForOutWhenUnconnected=off
  Orientation : Outport  Port=2  VectorParamsAs1DForOutWhenUnconnected=off
  Speed : Outport  Port=3  VectorParamsAs1DForOutWhenUnconnected=off
  V_Network_Out : Outport  Port=4  VectorParamsAs1DForOutWhenUnconnected=off
  wires:
  Vehicle Path Planner/1 -> Vehicle V2I Output/1
  Vehicle Sensors/1 -> Vehicle Path Planner/1
  Vehicle V2I Output/1 -> V_Network_Out/1
  Vehicle Sensors/2 -> Behavioural Planner/1
  Behavioural Planner/1 -> Longitudinal and Lateral Controllers/1(Speed Reference)
  Behavioural Planner/2 -> Longitudinal and Lateral Controllers/2(Inter Vehicular Distance)
  Behavioural Planner/3 -> Longitudinal and Lateral Controllers/3(Lead Speed)
  Behavioural Planner/4 -> Longitudinal and Lateral Controllers/4(drivingMode)
  Behavioural Planner/5 -> Longitudinal and Lateral Controllers/5(Dist2Stop)
  Transform to MOBATSim Coordinates/1(Position) -> Position/1
  Transform to MOBATSim Coordinates/2(Orientation) -> Orientation/1
  Vehicle Model - Kinematic 3DOF Single Track/2(xdot) -> Longitudinal and Lateral Controllers/7(Actual Speed), Speed/1
  Vehicle Model - Kinematic 3DOF Single Track/1(Pose) -> Longitudinal and Lateral Controllers/8(Actual Pose), Transform to MOBATSim Coordinates/1(Pose)
  Longitudinal and Lateral Controllers/1(ref Acc) -> Safety Filter/1(Reference Acceleration)
  Longitudinal and Lateral Controllers/2(ref Steering) -> Safety Filter/2(Reference Steering Angle)
  Safety Filter/1(Steering Angle Cmd) -> Vehicle Model - Kinematic 3DOF Single Track/1(WhlAngF)
  Safety Filter/2(Speed_input) -> Vehicle Model - Kinematic 3DOF Single Track/2(xdotin)
  Behavioural Planner/6 -> Longitudinal and Lateral Controllers/6(laneChange)

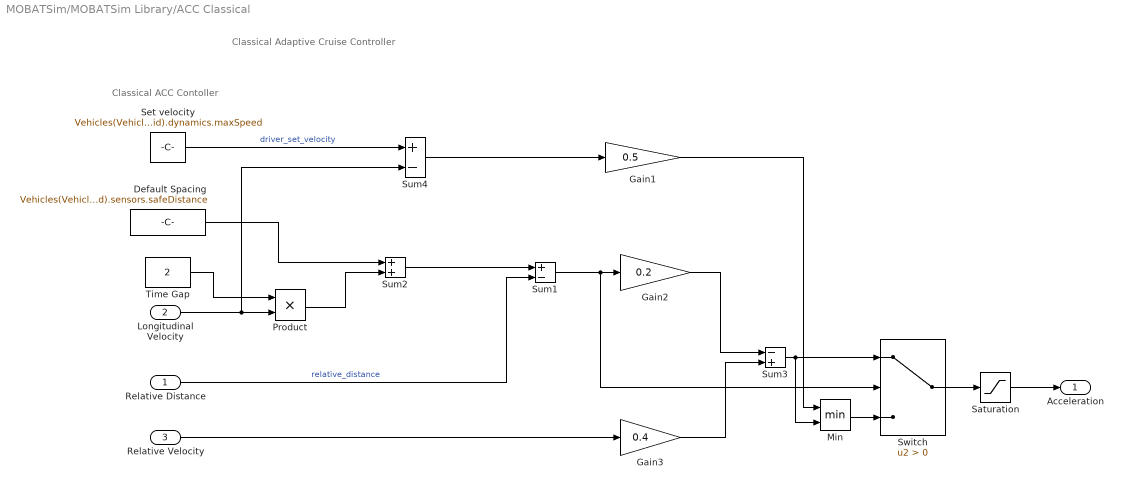
== system MOBATSim/MOBATSim Library/ACC Classical ==
  note: Classical ACC Contoller
  note: Classical Adaptive Cruise Controller
  Relative Distance : Inport
  Longitudinal Velocity : Inport  Port=2
  Relative Velocity : Inport  Port=3
  Default Spacing : Constant  Value=Vehicles(Vehicle_id).sensors.safeDistance  SampleTime=Sim_Ts
  Gain1 : Gain  Gain=0.5
  Gain2 : Gain  Gain=0.2
  Gain3 : Gain  Gain=0.4
  Min : MinMax  Inputs=2
  Product : Product
  Saturation : Saturate  UpperLimit=2  LowerLimit=-3
  Set velocity : Constant  Value=Vehicles(Vehicle_id).dynamics.maxSpeed  SampleTime=Sim_Ts
  Sum1 : Sum  Inputs=+-
  Sum2 : Sum
  Sum3 : Sum  Inputs=-+
  Sum4 : Sum  Inputs=+-
  Switch : Switch  Criteria=u2 > Threshold
  Time Gap : Constant  Value=2  SampleTime=Sim_Ts
  Acceleration : Outport  VectorParamsAs1DForOutWhenUnconnected=off
  wires:
  Longitudinal Velocity/1 -> Product/2, Sum4/2
  Default Spacing/1 -> Sum2/1
  Gain2/1 -> Sum3/1
  Sum4/1 -> Gain1/1
  Min/1 -> Switch/3
  Gain3/1 -> Sum3/2
  Switch/1 -> Saturation/1
  Relative Velocity/1 -> Gain3/1
  Time Gap/1 -> Product/1
  Saturation/1 -> Acceleration/1
  Product/1 -> Sum2/2
  Set velocity/1 -> Sum4/1  "driver_set_velocity"
  Sum3/1 -> Min/2, Switch/1
  Sum1/1 -> Switch/2, Gain2/1
  Gain1/1 -> Min/1
  Relative Distance/1 -> Sum1/2  "relative_distance"
  Sum2/1 -> Sum1/1

== system MOBATSim/MOBATSim Library/Platoon Controller - PID ==
  Inter Vehicular Distance : Inport
  Lead Speed : Inport  Port=2
  Vehicle Speed : Inport  Port=3
  Compare To Constant : simulink/Logic and Bit Operations/Compare To Constant  relop=>  const=2  OutDataTypeStr=uint8
  Constant : Constant  Value=meters
  Gain : Gain  Gain=1.4
  Multiport Switch : MultiPortSwitch  DataPortOrder=Zero-based contiguous  Inputs=2  zeroidx=on
  PID Controller5 : pid_lib/PID Controller  Controller=PID  Form=Parallel  TimeDomain=Continuous-time  UseExternalTs=off  SampleTime=-1  IntegratorMethod=Forward Euler  FilterMethod=Forward Euler  ControllerParametersSource=internal  P=2.0341199375219  I=0.0356576460366845  D=2.08363010404189  UseFilter=on  N=233.214579742572  TunerSelectOption=Transfer Function Based (PID Tuner App)  InitialConditionSource=internal  InitialConditionForIntegrator=0  InitialConditionForFilter=0  DifferentiatorICPrevScaledInput=0  ExternalReset=none  TrackingMode=off  Kt=1  LimitOutput=on  SatLimitsSource=internal  UpperSaturationLimit=100  LowerSaturationLimit=-100  LinearizeAsGain=on  AntiWindupMode=clamping  Kb=1  POutMin=[]  POutMax=[]  IOutMin=[]  IOutMax=[]  DOutMin=[]  DOutMax=[]  NOutMin=[]  NOutMax=[]  SumOutMin=[]  SumOutMax=[]  SaturationOutMin=[]  SaturationOutMax=[]  PParamMin=[]  PParamMax=[]  IParamMin=[]  IParamMax=[]  DParamMin=[]  DParamMax=[]  NParamMin=[]  NParamMax=[]  KbParamMin=[]  KbParamMax=[]  KtParamMin=[]  KtParamMax=[]  KbOutMin=[]  KbOutMax=[]  KtOutMin=[]  KtOutMax=[]  IntegratorOutMin=[]  IntegratorOutMax=[]  FilterOutMin=[]  FilterOutMax=[]  SumI1OutMin=[]  SumI1OutMax=[]  SumI2OutMin=[]  SumI2OutMax=[]  SumI3OutMin=[]  SumI3OutMax=[]  SumI4OutMin=[]  SumI4OutMax=[]  SumDOutMin=[]  SumDOutMax=[]  DifferentiatorOutMin=[]  DifferentiatorOutMax=[]  FilterDiffOutCoefMin=[]  FilterDiffOutCoefMax=[]  ReciprocalOutMin=[]  ReciprocalOutMax=[]  SumDenOutMin=[]  SumDenOutMax=[]  SumNumOutMin=[]  SumNumOutMax=[]  DivideOutMin=[]  DivideOutMax=[]  UdiffTsProdOutMin=[]  UdiffTsProdOutMax=[]  NTsProdOutMin=[]  NTsProdOutMax=[]  UintegralTsProdOutMin=[]  UintegralTsProdOutMax=[]  UngainTsProdOutMin=[]  UngainTsProdOutMax=[]  IntegratorContinuousStateAttributes=''  IntegratorStateMustResolveToSignalObject=off  IntegratorRTWStateStorageClass=Auto  FilterContinuousStateAttributes=''  FilterStateMustResolveToSignalObject=off  FilterRTWStateStorageClass=Auto  ParallelPVariant=InternalParameters  IdealPVariant=Disabled  IVariant=InternalParameters  DVariant=InternalParameters  IntegratorVariant=Continuous  SatVariant=Enabled  AWVariant=ContClampingParallel  PCopyVariant=Disabled  TRVariant=Disabled  FdbkBlocksVariant=Forward  IdealPFdbkVariant=Disabled  SatFdbkVariant=Disabled  DerivativeFilterVariant=ContFilter  NVariant=InternalParameters  NCopyVariant=Disabled  FilterICVariant=InternalICsFilter  IntegratorICVariant=InternalICs  ExternalResetVariant=Disabled  TRSumVariant=Passthrough  SumFdbkVariant=Disabled  SumVariant=Sum_PID  TsampFilterVariant=InternalTs  TsampNgainVariant=Passthrough  TsampIntegralVariant=Passthrough  ExternalSaturationOutDataTypeStr=Inherit: Same as second input
  Sum : Sum  Inputs=|-+
  Sum1 : Sum  Inputs=|++
  Sum2 : Sum  Inputs=|+-
  Transfer Fcn : TransferFcn  Numerator=[0.05]  Denominator=[1 2]
  ref speed : Outport  VectorParamsAs1DForOutWhenUnconnected=off
  wires:
  Transfer Fcn/1 -> PID Controller5/1
  Vehicle Speed/1 -> Gain/1, Sum/1
  PID Controller5/1 -> Multiport Switch/2
  Sum/1 -> Compare To Constant/1
  Multiport Switch/1 -> ref speed/1
  Compare To Constant/1 -> Multiport Switch/1
  Lead Speed/1 -> Sum/2, Multiport Switch/3
  Constant/1 -> Sum1/1
  Sum1/1 -> Sum2/2
  Gain/1 -> Sum1/2
  Sum2/1 -> Transfer Fcn/1
  Inter Vehicular Distance/1 -> Sum2/1

== system MOBATSim/MOBATSim Library/Pure Pursuit with Lane Changing ==
  Speed : Inport
  Pose : Inport  Port=2
  laneChange : Inport  Port=3
  MATLAB System1 : MATLABSystem  System=PurePursuit_WPGenerator  Vehicle_id=Vehicle_id  SimulateUsing=Interpreted execution
      mask Type: PurePursuit_WPGenerator
      mask Display:
      | image('MOBATSIM-Icon-Set_9- PurePursuit WP Generator.png');
      | port_label('input',1,'pose');
      | port_label('input',2,'speed');
      | port_label('input',3,'changeLane');
      | port_label('output',1,'nextWPs');
  Pure Pursuit : robotalgslib/Pure Pursuit  DesiredLinearVelocity=Vehicles(Vehicle_id).dynamics.maxSpeed  MaxAngularVelocity=1  LookaheadDistance=6  TargetDirPort=on  SimulateUsing=Code generation
  Terminator : Terminator
  Terminator1 : Terminator
  Wheel Steering Angle Formulation : Subsystem
  Reference Steering Angle : Outport
  wires:
  laneChange/1 -> MATLAB System1/3
  Speed/1 -> MATLAB System1/2
  Pose/1 -> Pure Pursuit/1, MATLAB System1/1
  Pure Pursuit/1 -> Terminator/1
  Pure Pursuit/2 -> Terminator1/1
  Pure Pursuit/3 -> Wheel Steering Angle Formulation/1(alpha)
  Wheel Steering Angle Formulation/1(referenceYawAngle) -> Reference Steering Angle/1
  MATLAB System1/1 -> Pure Pursuit/2

== system MOBATSim/MOBATSim Library/Stanley Lateral Control ==
  actualSpeed : Inport
  actualPose : Inport  Port=2
  laneChange : Inport  Port=3
  Constant5 : Constant
  Lateral Controller Stanley : drivingvehiclecontroller/Lateral Controller Stanley  ModelType=Kinematic bicycle model  PositionGainF=2.5  PositionGainR=2.5  YawRateGain=0.2  DelayGain=0.2  VehicleMass=1575  Lf=1.2  Lr=1.6  TireStiffness=19000  Wheelbase=3  MaxSteeringAngle=35
      settings: SourceProductBaseCode=DR
  MATLAB System : MATLABSystem  System=Stanley_RefPoseGenerator  Vehicle_id=Vehicle_id  SimulateUsing=Interpreted execution
      mask Type: Stanley_RefPoseGenerator
      mask Display:
      | image('MOBATSIM-Icon-Set_10- Stanley.png');
      | port_label('input',1,'pose');
      | port_label('input',2,'speed');
      | port_label('input',3,'changeLane');
      | port_label('output',1,'poseOut');
      | port_label('output',2,'referencePose');
  SteerCmd_Stanley : Outport
  wires:
  actualPose/1 -> MATLAB System/1
  MATLAB System/1 -> Lateral Controller Stanley/2
  actualSpeed/1 -> Lateral Controller Stanley/3, MATLAB System/2
  Constant5/1 -> Lateral Controller Stanley/4
  MATLAB System/2 -> Lateral Controller Stanley/1
  Lateral Controller Stanley/1 -> SteerCmd_Stanley/1
  laneChange/1 -> MATLAB System/3
